simulink model "TFlex_IFITC"  (R2018b)
settings: Solver=VariableStepAuto  StartTime=0.0  StopTime=t_end  RelTol=1e-3
values from neighbouring files (symbols this model uses):
  hyp = abs(hyp_sn(1:end-1))    [TFlex_IFITC_init.m]    (also in nlml_I_FITCv2.m = abs(hyp))
  Kuu = SEcov(u,u,hyp) + eye(Mu)*sn2    [nlml_I_FITCv2.m]
  Lu = chol(Kuu,'lower')    [nlml_I_FITCv2.m]
  Nkeep = 20    [TFlex_IFITC_init.m]
  sn = abs(hyp_sn(end))    [TFlex_IFITC_init.m]
  t_predict = 65    [TFlex_IFITC_init.m]
  ts = 1/1000    (= 0.001)    [TFlex_IFITC_init.m]
undefined symbols (not defined in the file or in its folder): a0, a1, a2, d_est, DiscIntNeverNeededParam, freqCogging, h, I_limit, k_est, Kd, Ki, Kp, LPden, LPnum, m_est, mu_u, P_estden, P_estnum, Pden, phaseCogging, Pnum, r, seed, sp_ts, svf_delay, tm, var_u
libraries: dspindex x6, simulink x5, dspfactors x2, dspmtrx3 x2
settings Model: Creator=wout7  LastModifiedBy=wout7

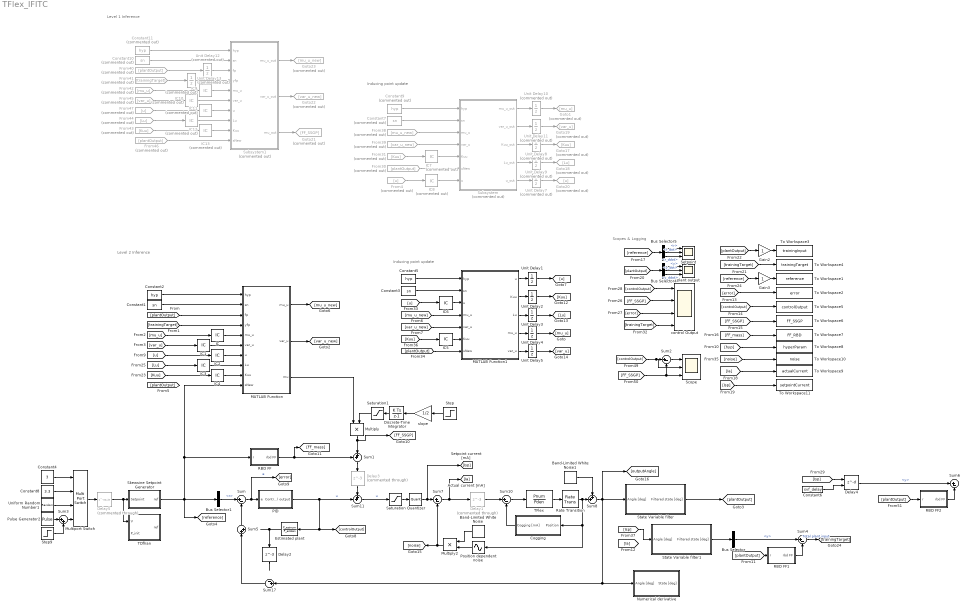
== system TFlex_IFITC ==
  note: Scopes & Logging
  note: Level 1 Inference
  note: Inducing point update
  note: Level 2 Inference
  note: Inducing point update
  Band-Limited White Noise : simulink/Sources/Band-Limited White Noise  Cov=[1e-3]  Ts=ts  seed=(seed+48124)
  Band-Limited White Noise1 : simulink/Sources/Band-Limited White Noise  Cov=[1e-15]  Ts=ts  seed=[23341]
  Bus Selector : BusSelector  OutputSignals=y
  Bus Selector1 : BusSelector  OutputSignals=r
  Bus Selector4 : BusSelector  OutputSignals=y,y_dot,y_ddot
  Bus Selector5 : BusSelector  OutputSignals=r,r_dot,r_ddot
  Cogging : Subsystem
  Constant1 : Constant  Value=sn  SampleTime=-1
  Constant10 : Constant  Commented=on  Value=sn  SampleTime=-1
  Constant11 : Constant  Commented=on  Value=hyp  SampleTime=-1
  Constant2 : Constant  Value=hyp  SampleTime=-1
  Constant3 : Constant  Value=sn  SampleTime=-1
  Constant4 : Constant  Value=3  SampleTime=sp_ts
  Constant5 : Constant  Value=hyp  SampleTime=-1
  Constant6 : Constant  Value=svf_delay  SampleTime=ts
  Constant7 : Constant  Commented=on  Value=sn  SampleTime=-1
  Constant8 : Constant  Value=3.3  SampleTime=sp_ts
  Constant9 : Constant  Commented=on  Value=hyp  SampleTime=-1
  Delay1 : Delay  Commented=through  DelayLength=3  InitialCondition=0
  Delay2 : Delay  DelayLength=3  InitialCondition=0
  Delay3 : Delay  Commented=through  DelayLength=3  InitialCondition=0
  Delay4 : Delay  DelayLengthSource=Input port  DelayLength=3  InitialCondition=0
      settings: InputPortMap=u0,p1
  Delay5 : Delay  Commented=through  DelayLength=sp_ts  SampleTime=sp_ts
  Discrete-Time Integrator : DiscreteIntegrator  SampleTime=-1  ICPrevOutput=DiscIntNeverNeededParam  ICPrevScaledInput=DiscIntNeverNeededParam
  Estimated plant : DiscreteTransferFcn  Numerator=P_estnum  Denominator=P_estden  SampleTime=ts
  From30 : From  Commented=on  GotoTag=plantOutput
  From31 : From  Commented=on  GotoTag=Kuu
  From38 : From  Commented=on  GotoTag=mu_u_new
  From39 : From  Commented=on  GotoTag=var_u_new
  From4 : From  Commented=on  GotoTag=u
  From40 : From  Commented=on  GotoTag=plantOutput
  From41 : From  Commented=on  GotoTag=trainingTarget
  From42 : From  Commented=on  GotoTag=mu_u
  From43 : From  Commented=on  GotoTag=Kuu
  From44 : From  Commented=on  GotoTag=Lu
  From45 : From  Commented=on  GotoTag=var_u
  From46 : From  Commented=on  GotoTag=plantOutput
  From47 : From  Commented=on  GotoTag=u
  Gain2 : Gain
  Gain3 : Gain
  Goto1 : Goto  Commented=on  GotoTag=mu_u
  Goto17 : Goto  Commented=on  GotoTag=Kuu
  Goto18 : Goto  Commented=on  GotoTag=Lu
  Goto19 : Goto  Commented=on  GotoTag=var_u
  Goto20 : Goto  Commented=on  GotoTag=u
  Goto21 : Goto  Commented=on  GotoTag=FF_SSGP
  Goto22 : Goto  Commented=on  GotoTag=var_u_new
  Goto23 : Goto  Commented=on  GotoTag=mu_u_new
  IC : InitialCondition  Value=mu_u
  IC1 : InitialCondition  Value=var_u
  IC10 : InitialCondition  Commented=on  Value=var_u
  IC11 : InitialCondition  Commented=on  Value=u
  IC12 : InitialCondition  Commented=on  Value=Lu
  IC13 : InitialCondition  Commented=on  Value=Kuu
  IC2 : InitialCondition  Value=u
  IC3 : InitialCondition  Value=Lu
  IC4 : InitialCondition  Value=Kuu
  IC5 : InitialCondition  Value=Kuu
  IC6 : InitialCondition  Value=u
  IC7 : InitialCondition  Commented=on  Value=Kuu
  IC8 : InitialCondition  Commented=on  Value=u
  IC9 : InitialCondition  Commented=on  Value=mu_u
  MATLAB Function : MATLAB Function  TreatAsAtomicUnit=on
  MATLAB Function1 : MATLAB Function  TreatAsAtomicUnit=on
  Multiply : Product
  Multiply2 : Product
  Multiport Switch : MultiPortSwitch
  Numerical derivative : Subsystem
  PID : Subsystem
  Position dependent noise : Sin  TimeSource=Use external signal  Amplitude=2.5  Bias=7.4979  Frequency=2*pi/13  SampleTime=0
  Pulse Generator2 : DiscretePulseGenerator  Amplitude=2*24  SampleTime=sp_ts
  Quantizer : Quantizer  QuantizationInterval=1
  RBD FF : Subsystem
  RBD FF1 : Subsystem
  RBD FF2 : Subsystem
  Rate Transition : RateTransition  OutPortSampleTime=ts
  Saturation : Saturate  UpperLimit=I_limit  LowerLimit=-I_limit
  Saturation1 : Saturate  UpperLimit=1  LowerLimit=0
  Scope : Scope  NumInputPorts=3
  Setpoint : Scope  NumInputPorts=3
  Skewsine Setpoint Generator : Subsystem
  State Variable filter : Subsystem
  State Variable filter1 : Subsystem
  Step : Step  Time=t_predict  SampleTime=0
  Step9 : Step  Time=0  After=-24  SampleTime=sp_ts
  Subsystem : Subsystem  Commented=on
  Subsystem1 : Subsystem  Commented=on
  Sum{,2,4,6..7,10} (6 alike) : Sum  Inputs=|+-
  Sum1 : Sum  Inputs=++|
  Sum11 : Sum  Inputs=++|
  Sum17 : Sum  Inputs=-+|
  Sum3 : Sum  Inputs=|++
  Sum5 : Sum  Inputs=|++
  Sum8 : Sum  Inputs=++|
  TDfhan : Subsystem
  TFlex : TransferFcn  Numerator=Pnum  Denominator=Pden  ContinuousStateAttributes='angle'
  To Workspace1 : ToWorkspace  VariableName=reference  SampleTime=-1
  To Workspace10 : ToWorkspace  VariableName=noise  SampleTime=-1
  To Workspace11 : ToWorkspace  VariableName=setpointCurrent  SampleTime=-1
  To Workspace2 : ToWorkspace  VariableName=error  SampleTime=-1
  To Workspace3 : ToWorkspace  VariableName=trainingInput  SampleTime=-1
  To Workspace4 : ToWorkspace  VariableName=trainingTarget  SampleTime=-1
  To Workspace5 : ToWorkspace  VariableName=controlOutput  SampleTime=-1
  To Workspace6 : ToWorkspace  VariableName=FF_SSGP  SampleTime=-1
  To Workspace7 : ToWorkspace  VariableName=FF_RBD  SampleTime=-1
  To Workspace8 : ToWorkspace  VariableName=hyperParam  SampleTime=-1
  To Workspace9 : ToWorkspace  VariableName=actualCurrent  SampleTime=-1
  Uniform Random Number1 : UniformRandomNumber  Minimum=-23  Maximum=23  Seed=seed  SampleTime=sp_ts
  Unit Delay{1..5} (5 alike) : UnitDelay  SampleTime=-1
  Unit Delay{7..13} (7 alike) : UnitDelay  Commented=on  SampleTime=-1
  control Output : Scope  NumInputPorts=4
  plant output : Scope  NumInputPorts=3
  slope : Gain  Gain=1/2
  wires:
  Sum/1 -> [error], PID/1(e)  "e"
  Sum5/1 -> Sum/2
  Bus Selector1/1 -> Sum/1  "<r>"
  [plantOutput] -> RBD FF1/1(r)
  TFlex/1 -> Rate Transition/1
  [reference] -> Gain3/1
  Bus Selector5/2 -> Setpoint/2  "<r_dot>"
  [FF_mass] -> To Workspace7/1
  Bus Selector5/1 -> Setpoint/1  "<r>"
  [error] -> To Workspace2/1
  Bus Selector5/3 -> Setpoint/3  "<r_ddot>"
  [controlOutput] -> To Workspace5/1
  [plantOutput] -> Gain2/1
  Gain2/1 -> To Workspace3/1
  [plantOutput] -> Bus Selector4/1
  Gain3/1 -> To Workspace1/1
  Bus Selector4/1 -> plant output/1  "<y>"
  Bus Selector4/3 -> plant output/3  "<y_ddot>"
  [reference] -> Bus Selector5/1
  [trainingTarget] -> To Workspace4/1
  Bus Selector4/2 -> plant output/2  "<y_dot>"
  [FF_SSGP] -> To Workspace6/1
  [trainingTarget] -> control Output/4
  [FF_SSGP] -> control Output/2
  [error] -> control Output/3
  [controlOutput] -> control Output/1
  [hyp] -> To Workspace8/1
  Sum4/1 -> [trainingTarget]  "Total plant input"
  Saturation/1 -> Quantizer/1
  PID/1(Control output) -> Estimated plant/1, [controlOutput], Sum11/2  "u"
  Estimated plant/1 -> Delay2/1
  Sum17/1 -> Sum5/1
  State Variable filter/1(Filtered state [deg]) -> [plantOutput]
  Rate Transition/1 -> Sum8/2, Cogging/1(Position), Position dependent noise/1
  Constant6/1 -> Delay4/2
  Sum11/1 -> Saturation/1  "u"
  [Isp] -> Delay4/1
  Sum8/1 -> [outputAngle], Sum17/2, Numerical derivative/1(Angle [deg]), State Variable filter/1(Angle [deg])
  Sum10/1 -> TFlex/1
  Delay2/1 -> ?
  RBD FF1/1(rbd FF) -> Sum4/2
  State Variable filter1/1(Filtered state [deg]) -> Bus Selector/1
  Sum7/1 -> Delay1/1, [Ia]
  Multiply2/1 -> Sum7/2, [noise]
  Cogging/1(Cogging [mA]) -> Sum10/2
  Quantizer/1 -> [Isp], Sum7/1
  Sum1/1 -> Delay3/1
  Delay3/1 -> Sum11/1
  Band-Limited White Noise/1 -> Multiply2/1
  Position dependent noise/1 -> Multiply2/2
  [noise] -> To Workspace10/1
  Pulse Generator2/1 -> Sum3/1
  Sum3/1 -> Multiport Switch/4
  Step9/1 -> Sum3/2
  Constant4/1 -> Multiport Switch/1
  Uniform Random Number1/1 -> Multiport Switch/3
  Constant8/1 -> Multiport Switch/2
  RBD FF/1(rbd FF) -> [FF_mass], Sum1/1
  [Ia] -> To Workspace9/1
  [Isp] -> To Workspace11/1
  Multiport Switch/1 -> Delay5/1
  Band-Limited White Noise1/1 -> Sum8/1
  Delay1/1 -> Sum10/1
  Delay5/1 -> TDfhan/1(V), Skewsine Setpoint Generator/1(Setpoint)
  [Isp] -> State Variable filter1/1(Angle [deg])
  Bus Selector/1 -> Sum4/1  "<y>"
  MATLAB Function/1(mu_u) -> [mu_u_new]
  MATLAB Function/2(var_u) -> [var_u_new]
  [mu_u] -> IC/1
  [var_u] -> IC1/1
  Constant1/1 -> MATLAB Function/2(sn)
  Constant2/1 -> MATLAB Function/1(hyp)
  Constant5/1 -> MATLAB Function1/1(hyp)
  Constant3/1 -> MATLAB Function1/2(sn)
  MATLAB Function1/1(u) -> Unit Delay1/1
  MATLAB Function1/2(Kuu) -> Unit Delay2/1
  MATLAB Function1/3(Lu) -> Unit Delay3/1
  [mu_u_new] -> MATLAB Function1/4("mu_u ")
  [var_u_new] -> MATLAB Function1/5("var_u ")
  [u] -> IC2/1
  [Kuu] -> IC4/1
  [Lu] -> IC3/1
  [plantOutput] -> MATLAB Function1/7(uNew)
  MATLAB Function1/4(mu_u) -> Unit Delay4/1
  MATLAB Function1/5(var_u) -> Unit Delay5/1
  [u] -> IC6/1
  [Kuu] -> IC5/1
  IC/1 -> MATLAB Function/5("mu_u ")
  IC1/1 -> MATLAB Function/6("var_u ")
  IC2/1 -> MATLAB Function/7(u)
  IC3/1 -> MATLAB Function/8(Lu)
  IC4/1 -> MATLAB Function/9(Kuu)
  IC5/1 -> MATLAB Function1/6("Kuu ")
  IC6/1 -> MATLAB Function1/3("u ")
  Unit Delay1/1 -> [u]
  Unit Delay2/1 -> [Kuu]
  Unit Delay3/1 -> [Lu]
  Unit Delay4/1 -> [mu_u]
  Unit Delay5/1 -> [var_u]
  [plantOutput] -> MATLAB Function/3(fp)
  [trainingTarget] -> MATLAB Function/4(yfp)
  Multiply/1 -> Sum1/2, [FF_SSGP]
  Saturation1/1 -> Multiply/2
  Discrete-Time Integrator/1 -> Saturation1/1
  slope/1 -> Discrete-Time Integrator/1
  Step/1 -> slope/1
  From31/1 -> IC7/1
  Unit Delay10/1 -> Goto1/1
  Unit Delay9/1 -> Goto18/1
  Unit Delay7/1 -> Goto20/1
  Unit Delay8/1 -> Goto17/1
  Constant9/1 -> Subsystem/1(hyp)
  Constant7/1 -> Subsystem/2(sn)
  From38/1 -> Subsystem/3(mu_u)
  From39/1 -> Subsystem/4(var_u)
  IC7/1 -> Subsystem/5(Kuu)
  From30/1 -> Subsystem/6(uNew)
  Subsystem/1(mu_u_out) -> Unit Delay10/1
  Unit Delay11/1 -> Goto19/1
  Subsystem/2(var_u_out) -> Unit Delay11/1
  Subsystem/3(Kuu_out) -> Unit Delay8/1
  Subsystem/4(Lu_out) -> Unit Delay9/1
  Subsystem/5(u_out) -> Unit Delay7/1
  From4/1 -> IC8/1
  IC8/1 -> Subsystem/7(u)
  From43/1 -> IC13/1
  From44/1 -> IC12/1
  From47/1 -> IC11/1
  From41/1 -> Unit Delay13/1
  From42/1 -> IC9/1
  From45/1 -> IC10/1
  From40/1 -> Unit Delay12/1
  Constant11/1 -> Subsystem1/1(hyp)
  Constant10/1 -> Subsystem1/2(sn)
  Unit Delay12/1 -> Subsystem1/3(fp)
  Unit Delay13/1 -> Subsystem1/4(yfp)
  IC9/1 -> Subsystem1/5(mu_u)
  IC10/1 -> Subsystem1/6(var_u)
  IC11/1 -> Subsystem1/7(u)
  IC12/1 -> Subsystem1/8(Lu)
  IC13/1 -> Subsystem1/9(Kuu)
  From46/1 -> Subsystem1/10(sNew)
  MATLAB Function/3(mu) -> Multiply/1
  Subsystem1/1(mu_u_out) -> Goto23/1
  Subsystem1/2(var_u_out) -> Goto22/1
  Subsystem1/3(mu_out) -> Goto21/1
  Skewsine Setpoint Generator/1(ref) -> RBD FF/1(r), MATLAB Function/10(sNew), [reference], Bus Selector1/1
  [controlOutput] -> Scope/2, Sum2/1
  [FF_SSGP] -> Scope/3, Sum2/2
  Sum2/1 -> Scope/1
  Delay4/1 -> Sum6/1  "<y>"
  RBD FF2/1(rbd FF) -> Sum6/2
  [plantOutput] -> RBD FF2/1(r)

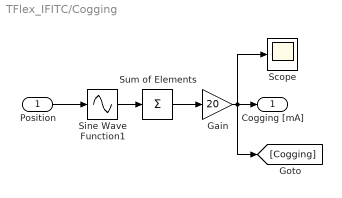
== system TFlex_IFITC/Cogging ==
  Position : Inport
  Gain : Gain  Gain=20
  Scope : Scope
  Sine Wave Function1 : Sin  TimeSource=Use external signal  Amplitude=ampCogging'  Frequency=2*pi./freqCogging'  Phase=phaseCogging'*2*pi  SampleTime=0
  Sum of Elements : Sum  Inputs=+
  Cogging [mA] : Outport
  wires:
  Gain/1 -> Scope/1, [Cogging], Cogging [mA]/1
  Sum of Elements/1 -> Gain/1
  Position/1 -> Sine Wave Function1/1
  Sine Wave Function1/1 -> Sum of Elements/1

== system TFlex_IFITC/Numerical derivative ==
  Angle [deg] : Inport
  Bus Creator : BusCreator  Inputs=3
  Discrete Derivative : simulink/Discrete/Discrete Derivative  gainval=1.0  ICPrevScaledInput=0.0  OutMin=[]  OutMax=[]  OutDataType=fixdt(1, 16)  OutScaling=2^-10  DoSatur=off
  Discrete Derivative1 : simulink/Discrete/Discrete Derivative  gainval=1.0  ICPrevScaledInput=0.0  OutMin=[]  OutMax=[]  OutDataType=fixdt(1, 16)  OutScaling=2^-10  DoSatur=off
  Numerical State : Scope  NumInputPorts=3
  State [deg] : Outport
  wires:
  Discrete Derivative/1 -> Numerical State/2, Bus Creator/2, Discrete Derivative1/1  "y_dot"
  Angle [deg]/1 -> Numerical State/1, Bus Creator/1, Discrete Derivative/1  "y"
  Bus Creator/1 -> State [deg]/1
  Discrete Derivative1/1 -> Numerical State/3, Bus Creator/3  "y_ddot"

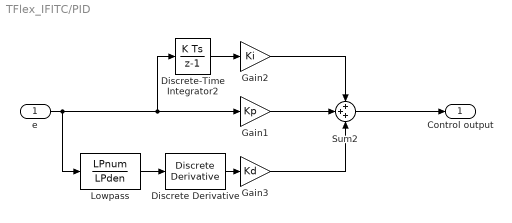
== system TFlex_IFITC/PID ==
  e : Inport
  Discrete Derivative : simulink/Discrete/Discrete Derivative  gainval=1.0  ICPrevScaledInput=0.0  OutMin=[]  OutMax=[]  OutDataType=fixdt(1, 16)  OutScaling=2^-10  DoSatur=off
  Discrete-Time Integrator2 : DiscreteIntegrator  SampleTime=-1  ICPrevOutput=DiscIntNeverNeededParam  ICPrevScaledInput=DiscIntNeverNeededParam
  Gain1 : Gain  Gain=Kp
  Gain2 : Gain  Gain=Ki
  Gain3 : Gain  Gain=Kd
  Lowpass : DiscreteTransferFcn  Numerator=LPnum  Denominator=LPden  SampleTime=ts
  Sum2 : Sum  Inputs=3
  Control output : Outport
  wires:
  Discrete-Time Integrator2/1 -> Gain2/1
  Gain1/1 -> Sum2/2
  Gain2/1 -> Sum2/1
  Gain3/1 -> Sum2/3
  Sum2/1 -> Control output/1
  e/1 -> Discrete-Time Integrator2/1, Gain1/1, Lowpass/1
  Lowpass/1 -> Discrete Derivative/1
  Discrete Derivative/1 -> Gain3/1

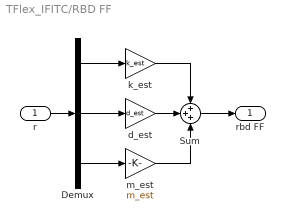
== system TFlex_IFITC/RBD FF ==
  r : Inport
  Demux : Demux  Outputs=3
  Sum : Sum  Inputs=+++
  d_est : Gain  Gain=d_est
  k_est : Gain  Gain=k_est
  m_est : Gain  Gain=m_est
  rbd FF : Outport
  wires:
  Demux/1 -> k_est/1
  Demux/2 -> d_est/1
  Demux/3 -> m_est/1
  m_est/1 -> Sum/3
  r/1 -> Demux/1
  d_est/1 -> Sum/2
  k_est/1 -> Sum/1
  Sum/1 -> rbd FF/1

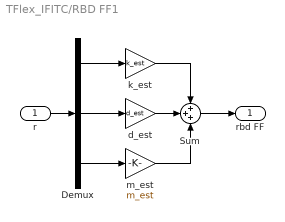
== system TFlex_IFITC/RBD FF1 ==
  r : Inport
  Demux : Demux  Outputs=3
  Sum : Sum  Inputs=+++
  d_est : Gain  Gain=d_est
  k_est : Gain  Gain=k_est
  m_est : Gain  Gain=m_est
  rbd FF : Outport
  wires:
  Demux/1 -> k_est/1
  Demux/2 -> d_est/1
  Demux/3 -> m_est/1
  m_est/1 -> Sum/3
  r/1 -> Demux/1
  d_est/1 -> Sum/2
  k_est/1 -> Sum/1
  Sum/1 -> rbd FF/1

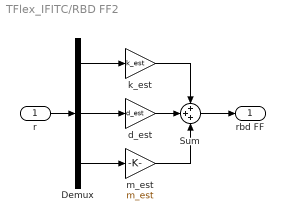
== system TFlex_IFITC/RBD FF2 ==
  r : Inport
  Demux : Demux  Outputs=3
  Sum : Sum  Inputs=+++
  d_est : Gain  Gain=d_est
  k_est : Gain  Gain=k_est
  m_est : Gain  Gain=m_est
  rbd FF : Outport
  wires:
  Demux/1 -> k_est/1
  Demux/2 -> d_est/1
  Demux/3 -> m_est/1
  m_est/1 -> Sum/3
  r/1 -> Demux/1
  d_est/1 -> Sum/2
  k_est/1 -> Sum/1
  Sum/1 -> rbd FF/1

== system TFlex_IFITC/Skewsine Setpoint Generator ==
  Setpoint : Inport
  Bus Creator : BusCreator  Inputs=3
  Delay : Delay  Commented=through  DelayLength=1  InitialCondition=0
  Subsystem : Subsystem
  ref : Outport
  wires:
  Subsystem/3(r_ddot) -> Bus Creator/3  "r_ddot"
  Bus Creator/1 -> ref/1
  Setpoint/1 -> Delay/1
  Subsystem/2(r_dot) -> Bus Creator/2  "r_dot"
  Subsystem/1(r) -> Bus Creator/1  "r"
  Delay/1 -> Subsystem/1(setpoint)

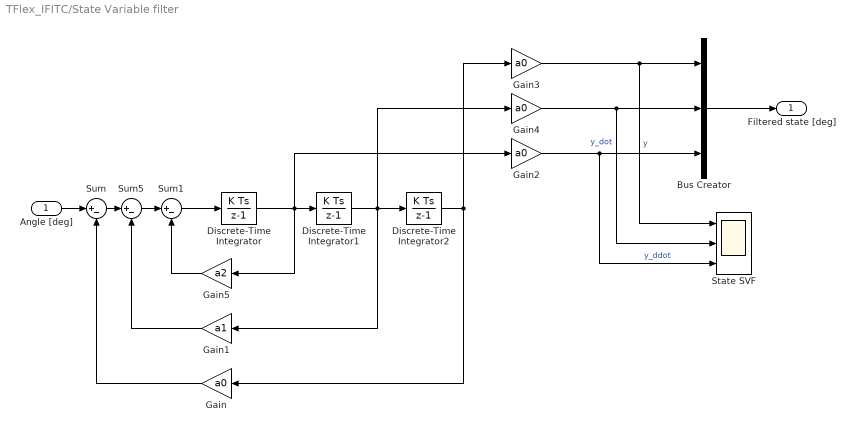
== system TFlex_IFITC/State Variable filter ==
  Angle [deg] : Inport
  Bus Creator : BusCreator  Inputs=3
  Discrete-Time Integrator : DiscreteIntegrator  SampleTime=-1  ICPrevOutput=DiscIntNeverNeededParam  ICPrevScaledInput=DiscIntNeverNeededParam
  Discrete-Time Integrator1 : DiscreteIntegrator  SampleTime=-1  ICPrevOutput=DiscIntNeverNeededParam  ICPrevScaledInput=DiscIntNeverNeededParam
  Discrete-Time Integrator2 : DiscreteIntegrator  SampleTime=-1  ICPrevOutput=DiscIntNeverNeededParam  ICPrevScaledInput=DiscIntNeverNeededParam
  Gain{,2..4} (4 alike) : Gain  Gain=a0
  Gain1 : Gain  Gain=a1
  Gain5 : Gain  Gain=a2
  State SVF : Scope  NumInputPorts=3
  Sum : Sum  Inputs=|+-
  Sum1 : Sum  Inputs=|+-
  Sum5 : Sum  Inputs=|+-
  Filtered state [deg] : Outport  SampleTime=ts
  wires:
  Bus Creator/1 -> Filtered state [deg]/1
  Sum1/1 -> Discrete-Time Integrator/1
  Angle [deg]/1 -> Sum/1
  Sum/1 -> Sum5/1
  Gain/1 -> Sum/2
  Gain1/1 -> Sum5/2
  Gain3/1 -> State SVF/1, Bus Creator/1  "y"
  Gain2/1 -> State SVF/3, Bus Creator/3  "y_ddot"
  Gain4/1 -> State SVF/2, Bus Creator/2  "y_dot"
  Gain5/1 -> Sum1/2
  Sum5/1 -> Sum1/1
  Discrete-Time Integrator/1 -> Discrete-Time Integrator1/1, Gain2/1, Gain5/1
  Discrete-Time Integrator1/1 -> Discrete-Time Integrator2/1, Gain4/1, Gain1/1
  Discrete-Time Integrator2/1 -> Gain3/1, Gain/1

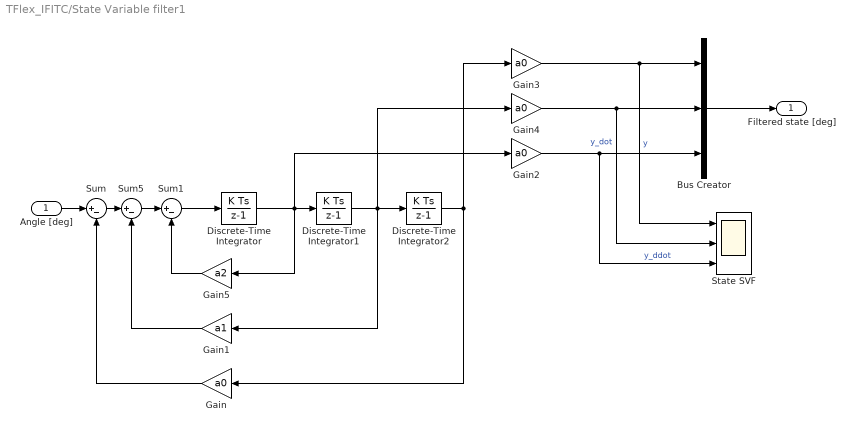
== system TFlex_IFITC/State Variable filter1 ==
  Angle [deg] : Inport
  Bus Creator : BusCreator  Inputs=3
  Discrete-Time Integrator : DiscreteIntegrator  SampleTime=-1  ICPrevOutput=DiscIntNeverNeededParam  ICPrevScaledInput=DiscIntNeverNeededParam
  Discrete-Time Integrator1 : DiscreteIntegrator  SampleTime=-1  ICPrevOutput=DiscIntNeverNeededParam  ICPrevScaledInput=DiscIntNeverNeededParam
  Discrete-Time Integrator2 : DiscreteIntegrator  SampleTime=-1  ICPrevOutput=DiscIntNeverNeededParam  ICPrevScaledInput=DiscIntNeverNeededParam
  Gain{,2..4} (4 alike) : Gain  Gain=a0
  Gain1 : Gain  Gain=a1
  Gain5 : Gain  Gain=a2
  State SVF : Scope  NumInputPorts=3
  Sum : Sum  Inputs=|+-
  Sum1 : Sum  Inputs=|+-
  Sum5 : Sum  Inputs=|+-
  Filtered state [deg] : Outport  SampleTime=ts
  wires:
  Bus Creator/1 -> Filtered state [deg]/1
  Sum1/1 -> Discrete-Time Integrator/1
  Angle [deg]/1 -> Sum/1
  Sum/1 -> Sum5/1
  Gain/1 -> Sum/2
  Gain1/1 -> Sum5/2
  Gain3/1 -> State SVF/1, Bus Creator/1  "y"
  Gain2/1 -> State SVF/3, Bus Creator/3  "y_ddot"
  Gain4/1 -> State SVF/2, Bus Creator/2  "y_dot"
  Gain5/1 -> Sum1/2
  Sum5/1 -> Sum1/1
  Discrete-Time Integrator/1 -> Discrete-Time Integrator1/1, Gain2/1, Gain5/1
  Discrete-Time Integrator1/1 -> Discrete-Time Integrator2/1, Gain4/1, Gain1/1
  Discrete-Time Integrator2/1 -> Gain3/1, Gain/1

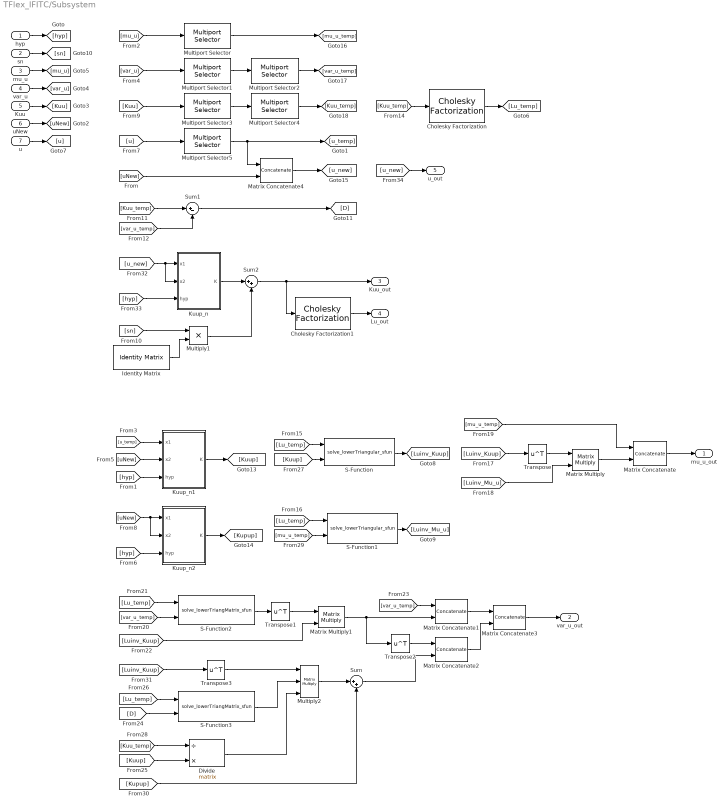
== system TFlex_IFITC/Subsystem ==
  hyp : Inport
  sn : Inport  Port=2
  mu_u : Inport  Port=3
  var_u : Inport  Port=4
  Kuu : Inport  Port=5
  uNew : Inport  Port=6
  u : Inport  Port=7
  Cholesky Factorization : dspfactors/Cholesky Factorization  errmode=Warning
      settings: SourceProductName=DSP System Toolbox  SourceProductBaseCode=DS
  Cholesky Factorization1 : dspfactors/Cholesky Factorization  errmode=Warning
      settings: SourceProductName=DSP System Toolbox  SourceProductBaseCode=DS
  Divide : Product  Inputs=/*  Multiplication=Matrix(*)
  Identity Matrix : dspmtrx3/Identity Matrix  Inherit=off  N=Nkeep+1  Ts=1  dataType=double  isSigned=on  wordLen=16  udDataType=sfix(16)  fracBitsMode=Best precision  numFracBits=15  OutDataTypeStr=double  LastOutDataTypeStr=double
      settings: SourceProductName=DSP System Toolbox
  Kuup_n : MATLAB Function  TreatAsAtomicUnit=on
  Kuup_n1 : MATLAB Function  TreatAsAtomicUnit=on
  Kuup_n2 : MATLAB Function  TreatAsAtomicUnit=on
  Matrix Concatenate : Concatenate  Mode=Multidimensional array
  Matrix Concatenate1 : Concatenate  Mode=Multidimensional array  ConcatenateDimension=2
  Matrix Concatenate2 : Concatenate  Mode=Multidimensional array  ConcatenateDimension=2
  Matrix Concatenate3 : Concatenate  Mode=Multidimensional array
  Matrix Concatenate4 : Concatenate  Mode=Multidimensional array
  Matrix Multiply : Product  Multiplication=Matrix(*)
  Matrix Multiply1 : Product  Multiplication=Matrix(*)
  Multiply1 : Product
  Multiply2 : Product  Inputs=3  Multiplication=Matrix(*)
  Multiport Selector{,1,3,5} (4 alike) : dspindex/Multiport Selector  rowsOrCols=Rows  idxCellArray={ 2:Nkeep+1}  idxErrMode=Clip Index
  Multiport Selector2 : dspindex/Multiport Selector  rowsOrCols=Columns  idxCellArray={ 2:Nkeep+1}  idxErrMode=Clip Index
  Multiport Selector4 : dspindex/Multiport Selector  rowsOrCols=Columns  idxCellArray={ 2:Nkeep+1}  idxErrMode=Clip Index
  S-Function : S-Function  FunctionName=solve_lowerTriangular_sfun  Parameters=Nkeep  SFunctionDeploymentMode=off  EnableBusSupport=off
  S-Function1 : S-Function  FunctionName=solve_lowerTriangular_sfun  Parameters=Nkeep  SFunctionDeploymentMode=off  EnableBusSupport=off
  S-Function2 : S-Function  FunctionName=solve_lowerTriangMatrix_sfun  Parameters=Nkeep  SFunctionDeploymentMode=off  EnableBusSupport=off
  S-Function3 : S-Function  FunctionName=solve_lowerTriangMatrix_sfun  Parameters=Nkeep  SFunctionDeploymentMode=off  EnableBusSupport=off
  Sum : Sum  Inputs=|++
  Sum1 : Sum  Inputs=|+-
  Sum2 : Sum  Inputs=|++
  Transpose{,1..3} (4 alike) : Math  Operator=transpose  SaturateOnIntegerOverflow=on
  mu_u_out : Outport
  var_u_out : Outport  Port=2
  Kuu_out : Outport  Port=3
  Lu_out : Outport  Port=4
  u_out : Outport  Port=5
  wires:
  Kuu/1 -> [Kuu]
  uNew/1 -> [uNew]
  hyp/1 -> [hyp]
  [hyp] -> Kuup_n1/3(hyp)
  [u_temp] -> Kuup_n1/1(x1)
  [uNew] -> Kuup_n1/2(x2)
  [uNew] -> Kuup_n2/2(x2), Kuup_n2/1(x1)
  [hyp] -> Kuup_n2/3(hyp)
  var_u/1 -> [var_u]
  mu_u/1 -> [mu_u]
  Cholesky Factorization/1 -> [Lu_temp]
  [Kuu_temp] -> Cholesky Factorization/1
  [Lu_temp] -> S-Function/1
  S-Function/1 -> [Luinv_Kuup]
  S-Function1/1 -> [Luinv_Mu_u]
  [Lu_temp] -> S-Function1/1
  Kuup_n2/1(K) -> [Kupup]
  [Luinv_Kuup] -> Transpose/1
  Transpose/1 -> Matrix Multiply/1
  [Luinv_Mu_u] -> Matrix Multiply/2
  Matrix Multiply/1 -> Matrix Concatenate/2
  [mu_u_temp] -> Matrix Concatenate/1
  Matrix Concatenate/1 -> mu_u_out/1
  [var_u_temp] -> S-Function2/2
  [Lu_temp] -> S-Function2/1
  S-Function2/1 -> Transpose1/1
  Transpose1/1 -> Matrix Multiply1/1
  [Luinv_Kuup] -> Matrix Multiply1/2
  Matrix Multiply1/1 -> Matrix Concatenate1/2, Transpose2/1
  [var_u_temp] -> Matrix Concatenate1/1
  Transpose2/1 -> Matrix Concatenate2/1
  Matrix Concatenate1/1 -> Matrix Concatenate3/1
  Matrix Concatenate2/1 -> Matrix Concatenate3/2
  [D] -> S-Function3/2
  [Lu_temp] -> S-Function3/1
  [Kuup] -> Divide/2
  [Kuu_temp] -> Divide/1
  Divide/1 -> Multiply2/3
  Kuup_n1/1(K) -> [Kuup]
  [Kuup] -> S-Function/2
  [mu_u_temp] -> S-Function1/2
  [Luinv_Kuup] -> Transpose3/1
  Transpose3/1 -> Multiply2/1
  Multiply2/1 -> Sum/1
  [Kupup] -> Sum/2
  Sum/1 -> Matrix Concatenate2/2
  Matrix Concatenate3/1 -> var_u_out/1
  Identity Matrix/1 -> Multiply1/2
  [sn] -> Multiply1/1
  Matrix Concatenate4/1 -> [u_new]
  [u_new] -> Kuup_n/2(x2), Kuup_n/1(x1)
  [hyp] -> Kuup_n/3(hyp)
  Multiply1/1 -> Sum2/2
  Kuup_n/1(K) -> Sum2/1
  Sum2/1 -> Kuu_out/1, Cholesky Factorization1/1
  Cholesky Factorization1/1 -> Lu_out/1
  [u_new] -> u_out/1
  S-Function3/1 -> Multiply2/2
  Multiport Selector5/1 -> [u_temp], Matrix Concatenate4/1
  [mu_u] -> Multiport Selector/1
  Multiport Selector/1 -> [mu_u_temp]
  [var_u] -> Multiport Selector1/1
  Multiport Selector1/1 -> Multiport Selector2/1
  Multiport Selector2/1 -> [var_u_temp]
  Multiport Selector4/1 -> [Kuu_temp]
  [Kuu] -> Multiport Selector3/1
  Multiport Selector3/1 -> Multiport Selector4/1
  u/1 -> [u]
  [u] -> Multiport Selector5/1
  [uNew] -> Matrix Concatenate4/2
  sn/1 -> [sn]
  [Kuu_temp] -> Sum1/1
  [var_u_temp] -> Sum1/2
  Sum1/1 -> [D]

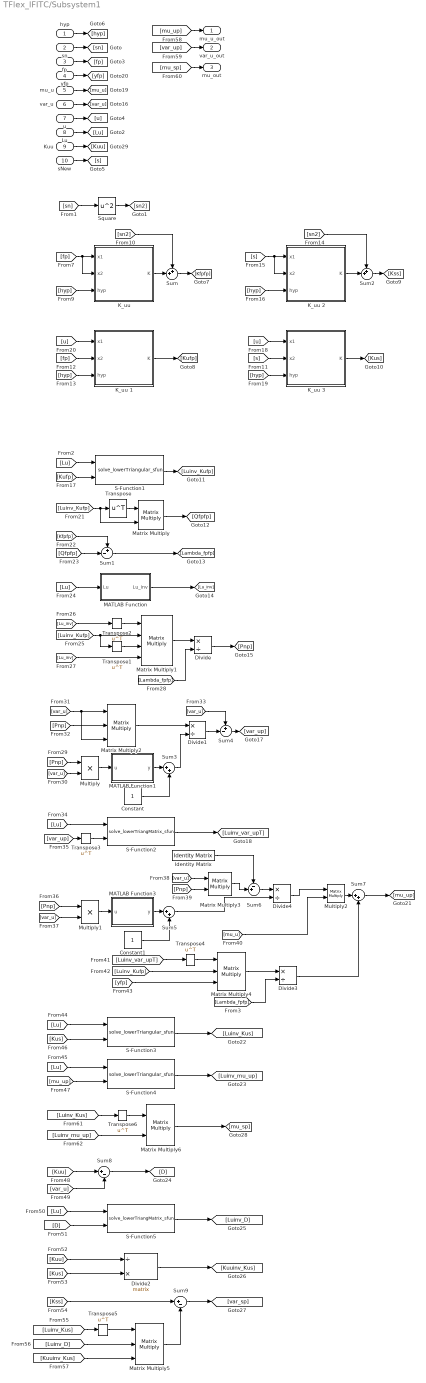
== system TFlex_IFITC/Subsystem1 ==
  hyp : Inport
  sn : Inport  Port=2
  fp : Inport  Port=3
  yfp : Inport  Port=4
  mu_u : Inport  Port=5
  var_u : Inport  Port=6
  u : Inport  Port=7
  Lu : Inport  Port=8
  Kuu : Inport  Port=9
  sNew : Inport  Port=10
  Constant : Constant
  Constant1 : Constant
  Divide{,1,3..4} (4 alike) : Product  Inputs=*/
  Divide2 : Product  Inputs=/*  Multiplication=Matrix(*)
  Identity Matrix : dspmtrx3/Identity Matrix  Inherit=off  N=Nkeep+1  Ts=1  dataType=double  isSigned=on  wordLen=16  udDataType=sfix(16)  fracBitsMode=Best precision  numFracBits=15  OutDataTypeStr=double  LastOutDataTypeStr=double
      settings: SourceProductName=DSP System Toolbox
  "K_uu " : MATLAB Function  TreatAsAtomicUnit=on
  K_uu 1 : MATLAB Function  TreatAsAtomicUnit=on
  K_uu 2 : MATLAB Function  TreatAsAtomicUnit=on
  K_uu 3 : MATLAB Function  TreatAsAtomicUnit=on
  MATLAB Function : MATLAB Function  TreatAsAtomicUnit=on
  MATLAB Function1 : MATLAB Function  TreatAsAtomicUnit=on
  MATLAB Function3 : MATLAB Function  TreatAsAtomicUnit=on
  Matrix Multiply : Product  Multiplication=Matrix(*)
  Matrix Multiply1 : Product  Inputs=4  Multiplication=Matrix(*)
  Matrix Multiply2 : Product  Inputs=3  Multiplication=Matrix(*)
  Matrix Multiply3 : Product  Multiplication=Matrix(*)
  Matrix Multiply4 : Product  Inputs=3  Multiplication=Matrix(*)
  Matrix Multiply5 : Product  Inputs=3  Multiplication=Matrix(*)
  Matrix Multiply6 : Product  Multiplication=Matrix(*)
  Multiply : Product
  Multiply1 : Product
  Multiply2 : Product  Multiplication=Matrix(*)
  S-Function1 : S-Function  FunctionName=solve_lowerTriangular_sfun  Parameters=Nkeep+1  SFunctionDeploymentMode=off  EnableBusSupport=off
  S-Function2 : S-Function  FunctionName=solve_lowerTriangMatrix_sfun  Parameters=Nkeep+1  SFunctionDeploymentMode=off  EnableBusSupport=off
  S-Function3 : S-Function  FunctionName=solve_lowerTriangular_sfun  Parameters=Nkeep+1  SFunctionDeploymentMode=off  EnableBusSupport=off
  S-Function4 : S-Function  FunctionName=solve_lowerTriangular_sfun  Parameters=Nkeep+1  SFunctionDeploymentMode=off  EnableBusSupport=off
  S-Function5 : S-Function  FunctionName=solve_lowerTriangMatrix_sfun  Parameters=Nkeep+1  SFunctionDeploymentMode=off  EnableBusSupport=off
  Square : Math  Operator=square  SaturateOnIntegerOverflow=on
  Sum : Sum  Inputs=++|
  Sum1 : Sum  Inputs=+-|
  Sum2 : Sum  Inputs=++|
  Sum3 : Sum  Inputs=|++
  Sum4 : Sum  Inputs=+-|
  Sum5 : Sum  Inputs=|++
  Sum6 : Sum  Inputs=-+|
  Sum7 : Sum  Inputs=|++
  Sum8 : Sum  Inputs=|+-
  Sum9 : Sum  Inputs=|+-
  Transpose{,1..6} (7 alike) : Math  Operator=transpose  SaturateOnIntegerOverflow=on
  mu_u_out : Outport
  var_u_out : Outport  Port=2
  mu_out : Outport  Port=3
  wires:
  yfp/1 -> [yfp]
  sn/1 -> [sn]
  Lu/1 -> [Lu]
  var_u/1 -> [var_u]
  [sn] -> Square/1
  Square/1 -> [sn2]
  fp/1 -> [fp]
  u/1 -> [u]
  sNew/1 -> [s]
  [fp] -> "K_uu "/2(x2), "K_uu "/1(x1)
  hyp/1 -> [hyp]
  [hyp] -> "K_uu "/3(hyp)
  "K_uu "/1(K) -> Sum/2
  [sn2] -> Sum/1
  Sum/1 -> [Kfpfp]
  [fp] -> K_uu 1/2(x2)
  [hyp] -> K_uu 1/3(hyp)
  K_uu 1/1(K) -> [Kufp]
  Sum2/1 -> [Kss]
  [s] -> K_uu 2/1(x1), K_uu 2/2(x2)
  [hyp] -> K_uu 2/3(hyp)
  [sn2] -> Sum2/1
  K_uu 2/1(K) -> Sum2/2
  K_uu 3/1(K) -> [Kus]
  [u] -> K_uu 3/1(x1)
  [hyp] -> K_uu 3/3(hyp)
  [u] -> K_uu 1/1(x1)
  [s] -> K_uu 3/2(x2)
  S-Function1/1 -> [Luinv_Kufp]
  [Lu] -> S-Function1/1
  [Kufp] -> S-Function1/2
  Transpose/1 -> Matrix Multiply/1
  [Luinv_Kufp] -> Transpose/1, Matrix Multiply/2
  Matrix Multiply/1 -> [Qfpfp]
  Sum1/1 -> [Lambda_fpfp]
  [Kfpfp] -> Sum1/1
  [Qfpfp] -> Sum1/2
  [Lu] -> MATLAB Function/1(Lu)
  MATLAB Function/1(Lu_inv) -> [Lu_inv]
  [Luinv_Kufp] -> Transpose1/1, Matrix Multiply1/2
  Transpose1/1 -> Matrix Multiply1/3
  [Lu_inv] -> Transpose2/1
  Transpose2/1 -> Matrix Multiply1/1
  [Lu_inv] -> Matrix Multiply1/4
  Matrix Multiply1/1 -> Divide/1
  [Lambda_fpfp] -> Divide/2
  Divide/1 -> [Pnp]
  [Pnp] -> Multiply/1
  [var_u] -> Multiply/2
  Multiply/1 -> MATLAB Function1/1(u)
  MATLAB Function1/1(y) -> Sum3/1
  Constant/1 -> Sum3/2
  [var_u] -> Matrix Multiply2/3, Matrix Multiply2/1
  [Pnp] -> Matrix Multiply2/2
  Matrix Multiply2/1 -> Divide1/1
  Sum3/1 -> Divide1/2
  Divide1/1 -> Sum4/2
  [var_u] -> Sum4/1
  Sum4/1 -> [var_up]
  S-Function2/1 -> [Luinv_var_upT]
  [Lu] -> S-Function2/1
  [var_up] -> Transpose3/1
  Transpose3/1 -> S-Function2/2
  [var_u] -> Multiply1/2
  [Pnp] -> Multiply1/1
  Multiply1/1 -> MATLAB Function3/1(u)
  MATLAB Function3/1(y) -> Sum5/1
  Constant1/1 -> Sum5/2
  Sum5/1 -> Divide4/2
  [var_u] -> Matrix Multiply3/1
  [Pnp] -> Matrix Multiply3/2
  mu_u/1 -> [mu_u]
  Identity Matrix/1 -> Sum6/1
  Matrix Multiply3/1 -> Sum6/2
  [mu_u] -> Multiply2/2
  Transpose4/1 -> Matrix Multiply4/1
  [Luinv_var_upT] -> Transpose4/1
  [Luinv_Kufp] -> Matrix Multiply4/2
  [yfp] -> Matrix Multiply4/3
  Multiply2/1 -> Sum7/1
  Divide3/1 -> Sum7/2
  Sum7/1 -> [mu_up]
  S-Function3/1 -> [Luinv_Kus]
  S-Function4/1 -> [Luinv_mu_up]
  [Lu] -> S-Function3/1
  [Lu] -> S-Function4/1
  [Kus] -> S-Function3/2
  [mu_up] -> S-Function4/2
  [Kuu] -> Sum8/1
  [var_u] -> Sum8/2
  Sum8/1 -> [D]
  S-Function5/1 -> [Luinv_D]
  [Lu] -> S-Function5/1
  [D] -> S-Function5/2
  Divide2/1 -> [Kuuinv_Kus]
  [Kuu] -> Divide2/1
  [Kus] -> Divide2/2
  Matrix Multiply5/1 -> Sum9/2
  [Kss] -> Sum9/1
  Sum9/1 -> [var_sp]
  [Luinv_Kus] -> Transpose5/1
  Transpose5/1 -> Matrix Multiply5/1
  [Luinv_D] -> Matrix Multiply5/2
  [Kuuinv_Kus] -> Matrix Multiply5/3
  [mu_up] -> mu_u_out/1
  [var_up] -> var_u_out/1
  Transpose6/1 -> Matrix Multiply6/1
  [Luinv_Kus] -> Transpose6/1
  [Luinv_mu_up] -> Matrix Multiply6/2
  Matrix Multiply6/1 -> [mu_sp]
  [mu_sp] -> mu_out/1
  Kuu/1 -> [Kuu]
  Matrix Multiply4/1 -> Divide3/1
  [Lambda_fpfp] -> Divide3/2
  Divide4/1 -> Multiply2/1
  Sum6/1 -> Divide4/1

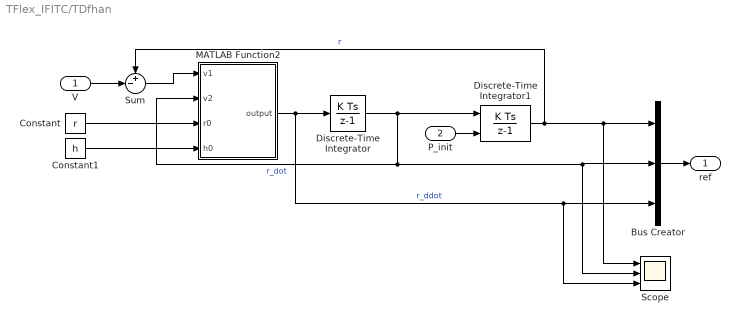
== system TFlex_IFITC/TDfhan ==
  V : Inport
  P_init : Inport  Port=2
  Bus Creator : BusCreator  Inputs=3
  Constant : Constant  Value=r  SampleTime=ts
  Constant1 : Constant  Value=h  SampleTime=ts
  Discrete-Time Integrator : DiscreteIntegrator  gainval=1  SampleTime=ts  ICPrevOutput=DiscIntNeverNeededParam  ICPrevScaledInput=DiscIntNeverNeededParam
  Discrete-Time Integrator1 : DiscreteIntegrator  gainval=1  InitialConditionSource=external  InitialCondition=-24  SampleTime=ts  ICPrevOutput=DiscIntNeverNeededParam  ICPrevScaledInput=DiscIntNeverNeededParam
  MATLAB Function2 : MATLAB Function  TreatAsAtomicUnit=on
  Scope : Scope  NumInputPorts=3
  Sum : Sum  Inputs=+-|
  ref : Outport
  wires:
  Sum/1 -> MATLAB Function2/1(v1)
  V/1 -> Sum/2
  Constant/1 -> MATLAB Function2/3(r0)
  Constant1/1 -> MATLAB Function2/4(h0)
  P_init/1 -> Discrete-Time Integrator1/2
  Discrete-Time Integrator1/1 -> Sum/1, Scope/1, Bus Creator/1  "r"
  Discrete-Time Integrator/1 -> Discrete-Time Integrator1/1, Scope/2, Bus Creator/2, MATLAB Function2/2(v2)  "r_dot"
  Bus Creator/1 -> ref/1
  MATLAB Function2/1(output) -> Scope/3, Bus Creator/3, Discrete-Time Integrator/1  "r_ddot"

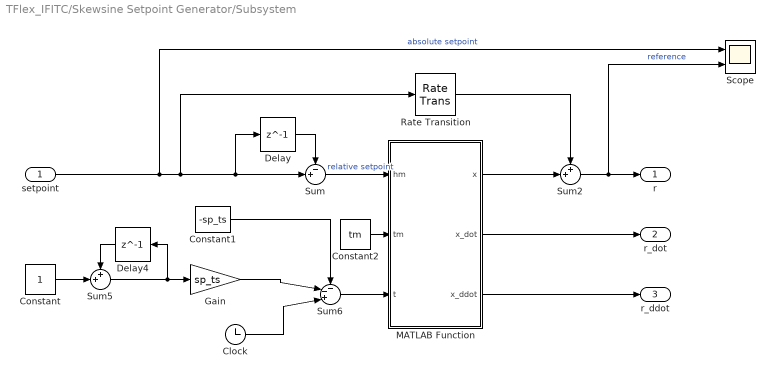
== system TFlex_IFITC/Skewsine Setpoint Generator/Subsystem ==
  setpoint : Inport
  Clock : Clock
      settings: Decimation=100
  Constant : Constant  SampleTime=sp_ts
  Constant1 : Constant  Value=-sp_ts  SampleTime=sp_ts
  Constant2 : Constant  Value=tm  SampleTime=sp_ts
  Delay : Delay  DelayLength=1  InitialCondition=0  SampleTime=sp_ts
  Delay4 : Delay  DelayLength=1  InitialCondition=0  SampleTime=sp_ts
  Gain : Gain  Gain=sp_ts
  MATLAB Function : MATLAB Function  TreatAsAtomicUnit=on
  Rate Transition : RateTransition  OutPortSampleTime=ts
  Scope : Scope  NumInputPorts=2
  Sum : Sum  Inputs=-+|
  Sum2 : Sum  Inputs=++|
  Sum5 : Sum  Inputs=++|
  Sum6 : Sum  Inputs=--+|
  r : Outport
  r_dot : Outport  Port=2
  r_ddot : Outport  Port=3
  wires:
  Delay4/1 -> Sum5/1
  Sum2/1 -> r/1, Scope/2  "reference"
  Sum5/1 -> Delay4/1, Gain/1
  Constant/1 -> Sum5/2
  MATLAB Function/3(x_ddot) -> r_ddot/1
  Clock/1 -> Sum6/3
  Delay/1 -> Sum/1
  Gain/1 -> Sum6/2
  Constant1/1 -> Sum6/1
  MATLAB Function/2(x_dot) -> r_dot/1
  Sum/1 -> MATLAB Function/1(hm)  "relative setpoint"
  Constant2/1 -> MATLAB Function/2(tm)
  Sum6/1 -> MATLAB Function/3(t)
  MATLAB Function/1(x) -> Sum2/2
  setpoint/1 -> Scope/1, Rate Transition/1, Delay/1, Sum/2  "absolute setpoint"
  Rate Transition/1 -> Sum2/1

== matlab function TFlex_IFITC/Subsystem/Kuup_n1 ==
  data: x1 input; K output size=[Nkeep,1]; x2 input; hyp input
function K = SquaredExpCov(x1,x2,hyp) %#codegen
coder.extrinsic('SEcov');
n = size(x1,1);
K = double(zeros(n,1));
K = SEcov(x1,x2,hyp);
end

== matlab function TFlex_IFITC/Skewsine Setpoint Generator/Subsystem/MATLAB Function ==
  settings: updateMethod=DISCRETE  sampleTime=ts
  data: hm input; x output; tm input; t input; x_dot output; x_ddot output
function [x,x_dot,x_ddot] = skewSine(hm,tm,t)

if (t>=0) && (t<=tm)
    x      = hm/tm*t - hm/(2*pi)*sin(2*pi/tm*t);
    x_dot  = hm/tm - hm/tm*cos(2*pi/tm*t);
    x_ddot = 2*pi*hm/(tm^2)*sin(2*pi/tm*t);
else
    x      = hm;
    x_dot  = 0;
    x_ddot = 0;
end

== matlab function TFlex_IFITC/MATLAB Function ==
  data: mu_u output; var_u output; hyp input size=[1,4]; sn input size=1; fp input size=[1,3]; yfp input size=[1]; mu_u input size=[Nkeep+1,1]; var_u input; u input; Lu input; Kuu input; mu output size=1; sNew input size=[1,3]
function [mu_u,var_u,mu] = I_FITC(hyp,sn,fp,yfp,mu_u,var_u,u,Lu,Kuu,sNew) %#codegen
coder.extrinsic('IncrementalFITC');
mu = double(1);
[mu, var ,mu_u,var_u] = IncrementalFITC(hyp,sn,u,sNew,fp,yfp,mu_u,var_u,Lu,Kuu);

== matlab function TFlex_IFITC/MATLAB Function1 ==
  data: hyp input; sn input; u input; u output; mu_u input; var_u input; Kuu input; uNew input size=[1,3]; Kuu output; Lu output; mu_u output; var_u output
function [u,Kuu,Lu,mu_u,var_u] = uUpdate(hyp,sn,u,mu_u,var_u,Kuu,uNew)%#codegen
coder.extrinsic('updateInducing');
Lu = double(zeros(size(Kuu)));
[u,Kuu,Lu,mu_u,var_u,Mu] = updateInducing(hyp,sn,u,mu_u,var_u,Kuu,uNew,0);

== matlab function TFlex_IFITC/Subsystem/Kuup_n2 ==
  data: x1 input; K output size=[1,1]; x2 input; hyp input
function K = SquaredExpCov(x1,x2,hyp) %#codegen
coder.extrinsic('SEcov');
K = double(1);
K = SEcov(x1,x2,hyp);
end

== matlab function TFlex_IFITC/TDfhan/MATLAB Function2 ==
  data: v1 input; output output; v2 input; r0 input; h0 input
function output = Fhan(v1,v2,r0, h0)
d = h0^2*r0;
a0 = h0*v2;
y = v1 + a0;
a1 = sqrt(d*(d+8*abs(y)));
a2 = a0 + sign(y)*(a1-d)/2;
sy = (sign(y+d)-sign(y-d))/2;
a = (a0+y-a2)*sy +a2;
sa = (sign(a+d)-sign(a-d))/2;
output = -r0 *(a/d -sign(a) )*sa - r0*sign(a);

== matlab function TFlex_IFITC/Subsystem1/K_uu  ==
  data: x1 input size=[1,3]; K output size=[1,1]; x2 input size=[1,3]; hyp input
function K = SquaredExpCov(x1,x2,hyp) %#codegen
coder.extrinsic('SEcov');
n = size(x1,1);
K = double(zeros(n,1));
K = SEcov(x1,x2,hyp);
end

== matlab function TFlex_IFITC/Subsystem/Kuup_n ==
  data: x1 input; K output size=[Nkeep+1,Nkeep+1]; x2 input; hyp input
function K = SquaredExpCov(x1,x2,hyp) %#codegen
coder.extrinsic('SEcov');
n = size(x1,1);
K = double(zeros(n));
K = SEcov(x1,x2,hyp);
end

== matlab function TFlex_IFITC/Subsystem1/K_uu 1 ==
  data: x1 input; K output size=[Nkeep+1,1]; x2 input; hyp input
function K = SquaredExpCov(x1,x2,hyp) %#codegen
coder.extrinsic('SEcov');
n = size(x1,1);
K = double(zeros(n,1));
K = SEcov(x1,x2,hyp);
end

== matlab function TFlex_IFITC/Subsystem1/K_uu 2 ==
  data: x1 input; K output size=[1,1]; x2 input; hyp input
function K = SquaredExpCov(x1,x2,hyp) %#codegen
coder.extrinsic('SEcov');
n = size(x1,1);
K = double(zeros(n,1));
K = SEcov(x1,x2,hyp);
end

== matlab function TFlex_IFITC/Subsystem1/K_uu 3 ==
  data: x1 input; K output size=[Nkeep+1,1]; x2 input; hyp input
function K = SquaredExpCov(x1,x2,hyp) %#codegen
coder.extrinsic('SEcov');
n = size(x1,1);
K = double(zeros(n,1));
K = SEcov(x1,x2,hyp);
end

== matlab function TFlex_IFITC/Subsystem1/MATLAB Function ==
  data: Lu input; Lu_inv output
function Lu_inv = inverse(Lu)
Lu_inv = inv(Lu);

== matlab function TFlex_IFITC/Subsystem1/MATLAB Function1 ==
  data: u input; y output
function y = Trace(u)
y = trace(u);

== matlab function TFlex_IFITC/Subsystem1/MATLAB Function3 ==
  data: u input; y output
function y = Trace(u)
y = trace(u);
